simulink model "modelLQR"  (R2015a)
settings: Solver=ode45  StartTime=0.0  StopTime=tsim  RelTol=1e-3
values from neighbouring files (symbols this model uses):
  A = [-R/L,0,0 ... (first row only)    [scriptadaptive.m]
  B = [1/L; 0; 0]    [scriptadaptive.m]
  Cy = [ 0,1,0]    [scriptadaptive.m]
  D = [0]    [scriptadaptive.m]
  gain = dcgain(syscd)    [script.m]    (also in scriptadaptive.m = Cy*inv( -(A-B*klq))*B)
  klq = lqrd(syscd.a,syscd.b,1*diag([1,1,1]), 100, zeros(3,1),1/200)    [script.m]    (also in scriptadaptive.m = lqr(sys,0.1*diag([1,1,1]), 1.5, zeros(3,1)))
undefined symbols (not defined in the file or in its folder): Continuous, Time
libraries: ctrlSharedLib x1
settings Model: Creator=dell  LastModifiedBy=user

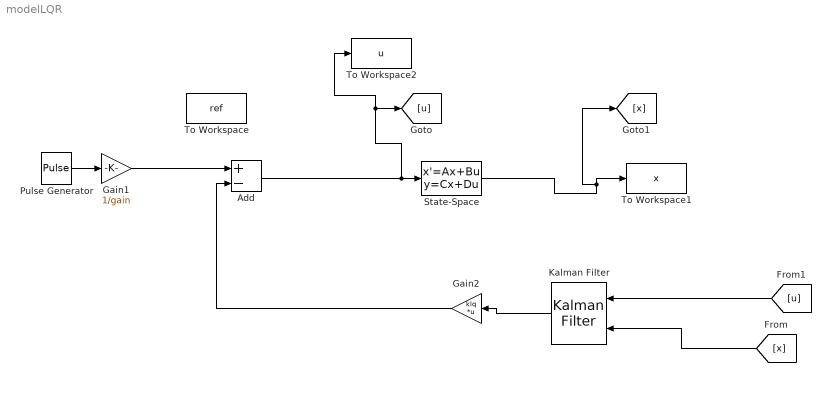
== system modelLQR ==
  Add : Sum  Inputs=+-
  Gain1 : Gain  Gain=1/gain
  Gain2 : Gain  Gain=klq  Multiplication=Matrix(K*u)
  Kalman Filter : ctrlSharedLib/Kalman Filter  TimeDomain=Continuous-Time  UseCurrentEstimator=on  ModelSource=Individual A, B, C, D matrices  ModelSourceVariable=ss(0.95,1,1,0,1)  A=A  B=B  C=Cy  D=D  NumberOfStates=1  NumberOfInputs=1  NumberOfOutputs=1  InitialEstimateSource=Dialog  X0=0  P0=10  UseK=off  UseGH=off  NumberOfProcessNoiseInputs=1  G=1  TimeInvariantG=on  H=0  TimeInvariantH=on  Q=0.000001  TimeInvariantQ=on  R=0.000001  TimeInvariantR=on  N=0  TimeInvariantN=on  AddInputPort=on  AddEnablePort=off  OutputEstimatedY=off  OutputP=off  Ts=1/200
  Pulse Generator : DiscretePulseGenerator  PulseType=Time based  Period=10  PulseWidth=50  PhaseDelay=5
  State-Space : StateSpace  A=A  B=B  C=Cy  D=D  X0=0
  To Workspace : ToWorkspace  VariableName=ref  SaveFormat=Timeseries  SampleTime=1/200
  To Workspace1 : ToWorkspace  VariableName=x  SaveFormat=Timeseries  SampleTime=1/200
  To Workspace2 : ToWorkspace  VariableName=u  SaveFormat=Timeseries  SampleTime=1/200
  wires:
  State-Space/1 -> [x], To Workspace1/1
  Add/1 -> State-Space/1, To Workspace2/1, [u]
  Pulse Generator/1 -> Gain1/1
  Kalman Filter/1 -> Gain2/1
  Gain1/1 -> Add/1
  [x] -> Kalman Filter/2
  [u] -> Kalman Filter/1
  Gain2/1 -> Add/2
